simulink subsystem "RackAndPinion"  (R2025a)
settings: Solver=VariableStepAuto  StartTime=0.0  StopTime=10.0  RelTol=1e-3
model mask{i_coef=0, J_pinion=0, m_rack=0, vis_friction_coef_rack=0}
settings Model: Creator=Глеб  LastModifiedBy=Глеб

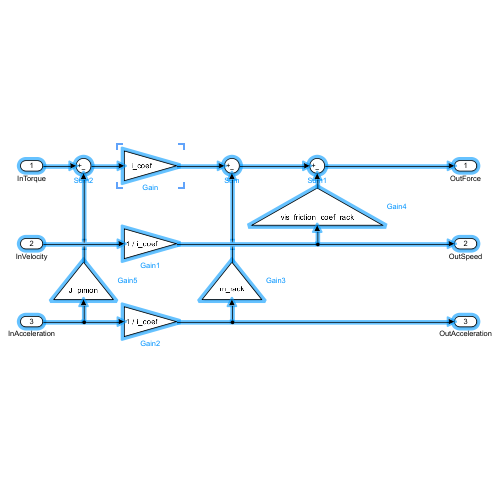
[thumbnail: Simulink's stored preview of the top-level diagram]
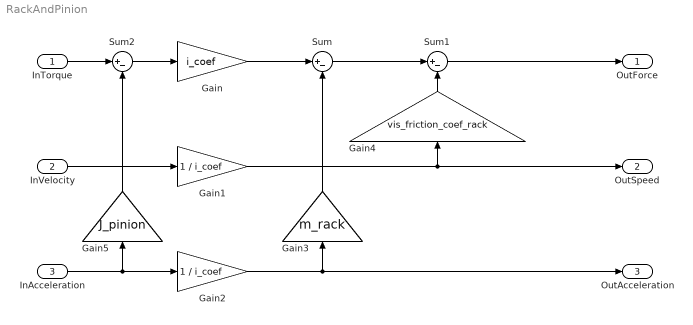
== system RackAndPinion ==
  InTorque : Inport
  InVelocity : Inport  Port=2
  InAcceleration : Inport  Port=3
  Gain : Gain  Gain=i_coef
  Gain1 : Gain  Gain=1 / i_coef
  Gain2 : Gain  Gain=1 / i_coef
  Gain3 : Gain  Gain=m_rack
  Gain4 : Gain  Gain=vis_friction_coef_rack
  Gain5 : Gain  Gain=J_pinion
  Sum : Sum  Inputs=|+-
  Sum1 : Sum  Inputs=|+-
  Sum2 : Sum  Inputs=|+-
  OutForce : Outport
  OutSpeed : Outport  Port=2
  OutAcceleration : Outport  Port=3
  wires:
  Gain/1 -> Sum/1
  Gain3/1 -> Sum/2
  Gain2/1 -> Gain3/1, OutAcceleration/1
  InVelocity/1 -> Gain1/1
  Gain5/1 -> Sum2/2
  InAcceleration/1 -> Gain5/1, Gain2/1
  Gain4/1 -> Sum1/2
  Sum2/1 -> Gain/1
  Sum1/1 -> OutForce/1
  Gain1/1 -> Gain4/1, OutSpeed/1
  InTorque/1 -> Sum2/1
  Sum/1 -> Sum1/1
